simulink library "pathFollowingCtrlAoATurb_cl"  (R2022a)
settings: Solver=VariableStepAuto  StartTime=0.0  StopTime=10.0  RelTol=1e-3
undefined symbols (not defined in the file): env, FLIGHTCONTROLLER, fltCtrl, initializeBussesFromBlock, pthCtrl1, vhcl
libraries: simulink x6, slpidlib x5, velocityAngle_ul x2, stopwatch_ul x1, courseFollowLookAhead_cl x1, ctrlAllocMatrix3Comp_cl x1, eulAng2RotMat_ul x1, angleBtw2Vecs_ul x1, vrlib x1, alphaBeta_ul x1, gnd2TanRotation_ul x1
settings Model: Creator=jldanie5  LastModifiedBy=jacob
settings SolverCC: AlgebraicLoopSolver=TrustRegion
settings DataIOCC: ReturnWorkspaceOutputs=off
settings DebuggingCC: UnconnectedInputMsg=warning  UnconnectedOutputMsg=warning  UnconnectedLineMsg=warning  SFMachineParentedDataDiag=warning  ArithmeticOperatorsInVariantConditions=warning
settings SFSimCC: CustomCodeUndefinedFunction=UseInterfaceOnly

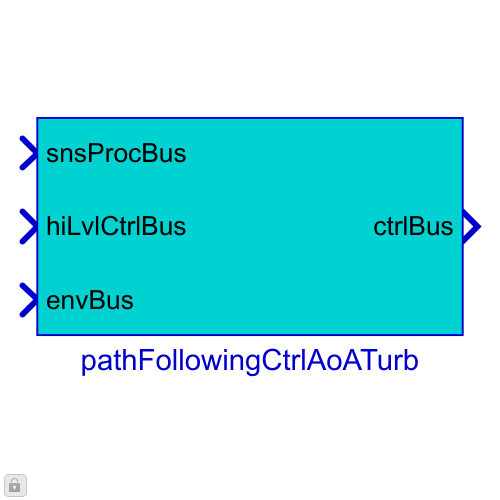
[thumbnail: Simulink's stored preview of the top-level diagram]
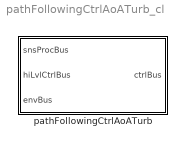
== system pathFollowingCtrlAoATurb_cl ==
  pathFollowingCtrlAoATurb : Subsystem  LoadFcn=initializeBussesFromBlock(gcb)  InitFcn=initializeBussesFromBlock(gcb)  StartFcn=initializeBussesFromBlock(gcb)  VariantControl=strcmpi(FLIGHTCONTROLLER,'pathFollowingControllerManta')  mask{initPosForInitSStar=vhcl.initPosVecGnd.Value, fluidDensity=env.water.density.Value, pathCtrl=pthCtrl1, aeroStruct=vhcl.struct('OCT.aeroSurf')}
      mask prompts: initPosForInitSStar "Initial Position"; fluidDensity "Fluid Density"; pathCtrl "Controller"; aeroStruct "Aerodynamic Structure"
      settings: MinAlgLoopOccurrences=on
      mask DialogControl Container3 Prompt: courseFollow Params
      mask DialogControl Container4 Prompt: setpointToOutput Params

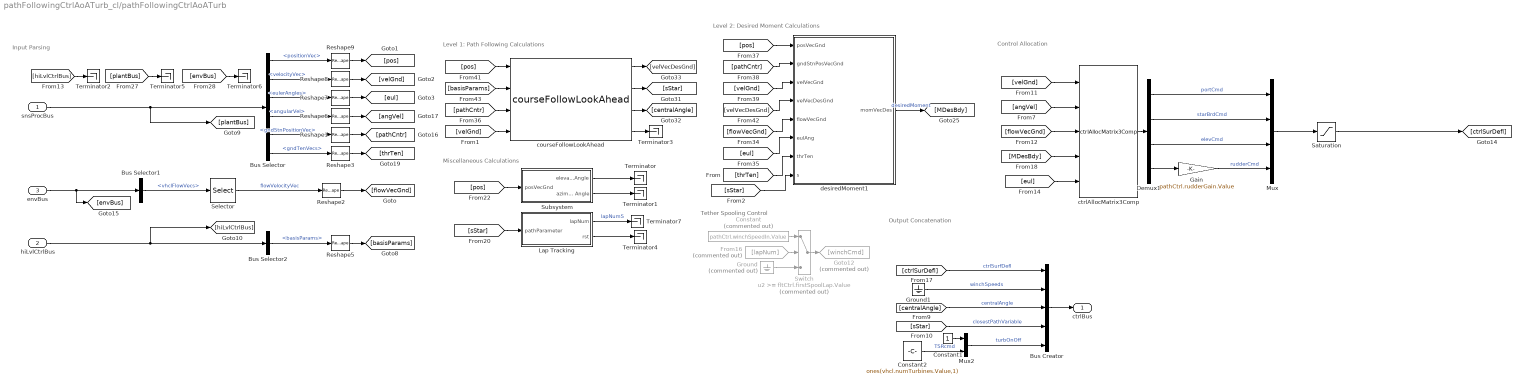
== system pathFollowingCtrlAoATurb_cl/pathFollowingCtrlAoATurb ==
  note: Control Allocation
  note: Miscellaneous Calculations
  note: Output Concatenation
  note: Tether Spooling Control
  note: Input Parsing
  note: Level 1: Path Following Calculations
  note: Level 2: Desired Moment Calculations
  snsProcBus : Inport  OutDataTypeStr=Bus: sensorsProcessingBus
  hiLvlCtrlBus : Inport  Port=2  OutDataTypeStr=Bus: hiLvlCtrlBus
  envBus : Inport  Port=3  OutDataTypeStr=Bus: envBus
  Bus Creator : BusCreator  Inputs=5
  Bus Selector : BusSelector  OutputSignals=positionVec,velocityVec,eulerAngles,angularVel,gndStnPositionVec,gndTenVecs
  Bus Selector1 : BusSelector  OutputSignals=vhclFlowVecs
  Bus Selector2 : BusSelector  OutputSignals=basisParams
  Constant : Constant  Commented=on  Value=pathCtrl.winchSpeedIn.Value
  Constant1 : Constant
  Constant2 : Constant  Value=ones(vhcl.numTurbines.Value,1)
  Demux1 : Demux
  From16 : From  Commented=on  GotoTag=lapNum
  Gain : Gain  Gain=pathCtrl.rudderGain.Value
  Goto12 : Goto  Commented=on  GotoTag=winchCmd
  Ground : Ground  Commented=on
  Ground1 : Ground
  Lap Tracking : Subsystem
  Mux : Mux
  Mux2 : Mux  Inputs=2
  Reshape{1..3,5..9} (8 alike) : Reshape  OutputDimensionality=Column vector (2-D)
  Saturation : Saturate  UpperLimit=30  LowerLimit=-30
  Selector : Selector  NumberOfDimensions=2  InputPortWidth=3  IndexOptions=Select all,Index vector (dialog)  Indices=[1 3],5  OutputSizes=1,1
  Subsystem : Subsystem
  Switch : Switch  Commented=on  Threshold=fltCtrl.firstSpoolLap.Value  SaturateOnIntegerOverflow=off  InputSameDT=off
  Terminator{,1..7} (8 alike) : Terminator
  courseFollowLookAhead : courseFollowLookAhead_cl/courseFollowLookAhead  SystemSampleTime=-1  VariantActivationTime=update diagram  Latency=0  AutoFrameSizeCalculation=off
  ctrlAllocMatrix3Comp : ctrlAllocMatrix3Comp_cl/ctrlAllocMatrix3Comp  aeroStruct=vhcl.struct('OCT.aeroSurf')  fluidDensity=fluidDensity  arms=vhcl.struct('OCT.thrAttch')
  desiredMoment1 : Subsystem
  ctrlBus : Outport  OutDataTypeStr=Bus: fltCtrlBus  VectorParamsAs1DForOutWhenUnconnected=off
  wires:
  Bus Selector/6 -> Reshape3/1  "<gndTenVecs>"
  Reshape3/1 -> [thrTen]
  snsProcBus/1 -> [plantBus], Bus Selector/1
  Bus Selector/2 -> Reshape8/1  "<velocityVec>"
  Bus Selector/1 -> Reshape9/1  "<positionVec>"
  Bus Selector/3 -> Reshape7/1  "<eulerAngles>"
  Bus Creator/1 -> ctrlBus/1
  Ground1/1 -> Bus Creator/2  "winchSpeeds"
  hiLvlCtrlBus/1 -> [hiLvlCtrlBus], Bus Selector2/1
  [centralAngle] -> Bus Creator/3  "centralAngle"
  [sStar] -> Bus Creator/4  "closestPathVariable"
  Bus Selector/4 -> Reshape6/1  "<angularVel>"
  [angVel] -> ctrlAllocMatrix3Comp/2
  [velGnd] -> ctrlAllocMatrix3Comp/1
  [flowVecGnd] -> ctrlAllocMatrix3Comp/3
  Demux1/1 -> Mux/1  "portCmd"
  Demux1/2 -> Mux/2  "starBrdCmd"
  [MDesBdy] -> ctrlAllocMatrix3Comp/4
  [ctrlSurDefl] -> Bus Creator/1  "ctrlSurfDefl"
  Bus Selector2/1 -> Reshape5/1  "<basisParams>"
  Reshape5/1 -> [basisParams]
  Reshape2/1 -> [flowVecGnd]
  Reshape6/1 -> [angVel]
  Reshape7/1 -> [eul]
  Reshape8/1 -> [velGnd]
  Reshape9/1 -> [pos]
  [eul] -> ctrlAllocMatrix3Comp/5
  Selector/1 -> Reshape2/1  "flowVelocityVec"
  envBus/1 -> [envBus], Bus Selector1/1
  Bus Selector1/1 -> Selector/1  "<vhclFlowVecs>"
  Reshape1/1 -> [pathCntr]
  Bus Selector/5 -> Reshape1/1  "<gndStnPositionVec>"
  Demux1/4 -> Gain/1
  [pos] -> Subsystem/1(posVecGnd)
  Subsystem/1(elevationAngle) -> Terminator/1
  Subsystem/2(azimuth Angle) -> Terminator1/1
  [sStar] -> Lap Tracking/1(pathParameter)
  Lap Tracking/2(rst) -> Terminator4/1
  Lap Tracking/1(lapNum) -> Terminator7/1  "lapNumS"
  [plantBus] -> Terminator5/1
  [envBus] -> Terminator6/1
  Switch/1 -> Goto12/1
  From16/1 -> Switch/2
  Constant/1 -> Switch/1
  Ground/1 -> Switch/3
  ctrlAllocMatrix3Comp/1 -> Demux1/1
  Gain/1 -> Mux/4  "rudderCmd"
  [hiLvlCtrlBus] -> Terminator2/1
  Mux2/1 -> Bus Creator/5  "turbOnOff"
  Constant1/1 -> Mux2/1
  Constant2/1 -> Mux2/2  "TSRcmd"
  [velVecDesGnd] -> desiredMoment1/4(velVecDesGnd)
  [velGnd] -> desiredMoment1/3(velVecGnd)
  [eul] -> desiredMoment1/6(eulAng)
  [basisParams] -> courseFollowLookAhead/2
  [pathCntr] -> desiredMoment1/2(gndStnPosVecGnd)
  courseFollowLookAhead/2 -> [sStar]
  [pos] -> desiredMoment1/1(posVecGnd)
  [pathCntr] -> courseFollowLookAhead/3
  desiredMoment1/1(momVecDes) -> [MDesBdy]  "desiredMoment"
  [pos] -> courseFollowLookAhead/1
  courseFollowLookAhead/3 -> [centralAngle]
  courseFollowLookAhead/4 -> Terminator3/1
  courseFollowLookAhead/1 -> [velVecDesGnd]
  [flowVecGnd] -> desiredMoment1/5(flowVecGnd)
  [thrTen] -> desiredMoment1/7(thrTen)
  [velGnd] -> courseFollowLookAhead/4
  Saturation/1 -> [ctrlSurDefl]
  Mux/1 -> Saturation/1
  Demux1/3 -> Mux/3  "elevCmd"
  [sStar] -> desiredMoment1/8(s)

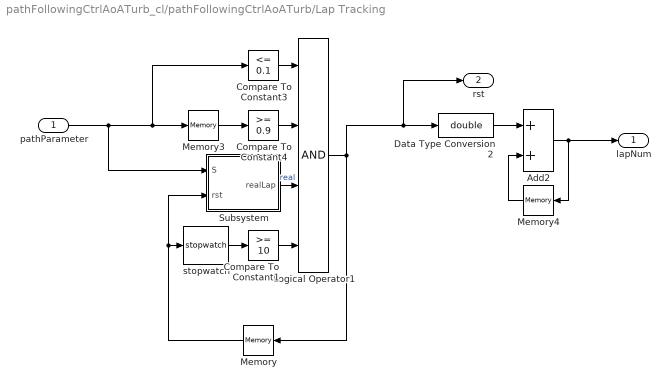
== system pathFollowingCtrlAoATurb_cl/pathFollowingCtrlAoATurb/Lap Tracking ==
  pathParameter : Inport
  Add2 : Sum
  Compare To Constant1 : simulink/Logic and Bit Operations/Compare To Constant  relop=>=  const=10  OutDataTypeStr=boolean
  Compare To Constant3 : simulink/Logic and Bit Operations/Compare To Constant  relop=<=  const=0.1  OutDataTypeStr=boolean
  Compare To Constant4 : simulink/Logic and Bit Operations/Compare To Constant  relop=>=  const=0.9  OutDataTypeStr=boolean
  Data Type Conversion2 : DataTypeConversion  OutDataTypeStr=double  SaturateOnIntegerOverflow=off  RndMeth=Floor
  Logical Operator1 : Logic  Inputs=4  AllPortsSameDT=off  OutDataTypeStr=boolean
  Memory : Memory  InitialCondition=false
  Memory3 : Memory
  Memory4 : Memory
  Subsystem : Subsystem
  stopwatch : stopwatch_ul/stopwatch  SystemSampleTime=-1  VariantActivationTime=update diagram  Latency=0  AutoFrameSizeCalculation=off
  lapNum : Outport  VectorParamsAs1DForOutWhenUnconnected=off
  rst : Outport  Port=2  VectorParamsAs1DForOutWhenUnconnected=off
  wires:
  Compare To Constant3/1 -> Logical Operator1/1
  Memory3/1 -> Compare To Constant4/1
  Data Type Conversion2/1 -> Add2/1
  Logical Operator1/1 -> rst/1, Data Type Conversion2/1, Memory/1
  Memory4/1 -> Add2/2
  Add2/1 -> lapNum/1, Memory4/1
  Compare To Constant4/1 -> Logical Operator1/2
  pathParameter/1 -> Subsystem/1(S), Compare To Constant3/1, Memory3/1
  stopwatch/1 -> Compare To Constant1/1
  Memory/1 -> Subsystem/2(rst), stopwatch/1
  Compare To Constant1/1 -> Logical Operator1/4
  Subsystem/1(realLap) -> Logical Operator1/3  "real"

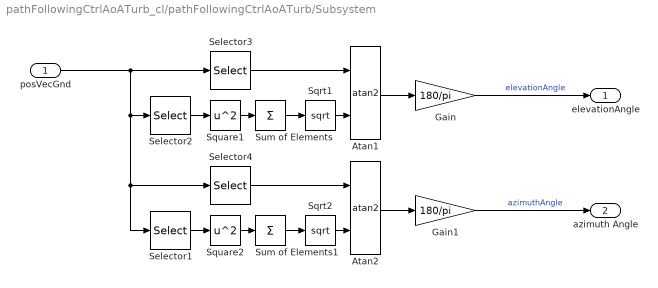
== system pathFollowingCtrlAoATurb_cl/pathFollowingCtrlAoATurb/Subsystem ==
  posVecGnd : Inport
  Atan1 : Trigonometry  Operator=atan2
  Atan2 : Trigonometry  Operator=atan2
  Gain : Gain  Gain=180/pi
  Gain1 : Gain  Gain=180/pi
  Selector1 : Selector  InputPortWidth=3  IndexOptions=Index vector (dialog)  Indices=1  OutputSizes=1
  Selector2 : Selector  InputPortWidth=3  IndexOptions=Index vector (dialog)  Indices=[1 2]  OutputSizes=1
  Selector3 : Selector  InputPortWidth=3  IndexOptions=Index vector (dialog)  Indices=3  OutputSizes=1
  Selector4 : Selector  InputPortWidth=3  IndexOptions=Index vector (dialog)  Indices=2  OutputSizes=1
  Sqrt1 : Sqrt
  Sqrt2 : Sqrt
  Square1 : Math  Operator=square  SignedPower=on
  Square2 : Math  Operator=square  SignedPower=on
  Sum of Elements : Sum  Inputs=+
  Sum of Elements1 : Sum  Inputs=+
  elevationAngle : Outport
  azimuth Angle : Outport  Port=2
  wires:
  Sqrt1/1 -> Atan1/2
  Square1/1 -> Sum of Elements/1
  Selector3/1 -> Atan1/1
  Sum of Elements/1 -> Sqrt1/1
  Atan1/1 -> Gain/1
  Selector2/1 -> Square1/1
  Gain/1 -> elevationAngle/1  "elevationAngle"
  Atan2/1 -> Gain1/1
  Square2/1 -> Sum of Elements1/1
  Sum of Elements1/1 -> Sqrt2/1
  Selector1/1 -> Square2/1
  posVecGnd/1 -> Selector1/1, Selector4/1, Selector2/1, Selector3/1
  Sqrt2/1 -> Atan2/2
  Selector4/1 -> Atan2/1
  Gain1/1 -> azimuth Angle/1  "azimuthAngle"

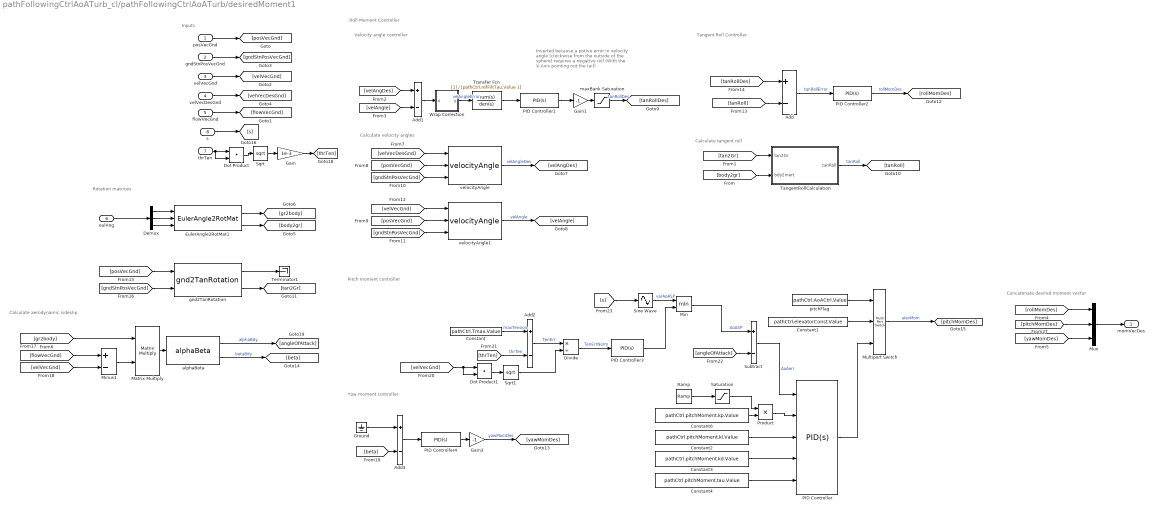
== system pathFollowingCtrlAoATurb_cl/pathFollowingCtrlAoATurb/desiredMoment1 ==
  note: Roll Moment Controller
  note: Calculate aerodynamic sideslip
  note: Concatenate desired moment vector
  note: Tangent Roll Controller
  note: Calculate tangent roll
  note: Calculate velocity angles
  note: Rotation matrices
  note: Inputs
  note: Velocity angle controller
  note: Inverted because a potive error
      | in velocity angle (clockwise from the
      | outside of the sphere) requires a negative
      | roll (With the X-Axis pointing out the tail)
  note: Pitch moment controller
  note: Yaw moment controller
  posVecGnd : Inport
  gndStnPosVecGnd : Inport  Port=2
  velVecGnd : Inport  Port=3
  velVecDesGnd : Inport  Port=4
  flowVecGnd : Inport  Port=5
  eulAng : Inport  Port=6
  thrTen : Inport  Port=7
  s : Inport  Port=8
  Add{,1..3} (4 alike) : Sum  Inputs=+-
  Constant : Constant  Value=pathCtrl.Tmax.Value
  Constant1 : Constant  Value=pathCtrl.elevatorConst.Value
  Constant2 : Constant  Value=pathCtrl.pitchMoment.ki.Value
  Constant3 : Constant  Value=pathCtrl.pitchMoment.kd.Value
  Constant4 : Constant  Value=pathCtrl.pitchMoment.tau.Value
  Constant6 : Constant  Value=pathCtrl.pitchMoment.kp.Value
  Demux : Demux  Outputs=3
  Divide : Product  Inputs=*/
  Dot Product : DotProduct  OutDataTypeStr=Inherit: Inherit via internal rule
  Dot Product1 : DotProduct  OutDataTypeStr=Inherit: Inherit via internal rule
  EulerAngle2RotMat1 : eulAng2RotMat_ul/EulerAngle2RotMat  SystemSampleTime=-1  VariantActivationTime=update diagram  Latency=0  AutoFrameSizeCalculation=off
  Gain : Gain  Gain=1e-3
  Gain1 : Gain  Gain=-1
  Gain3 : Gain  Gain=-1
  Ground : Ground
  Matrix Multiply : Product  Multiplication=Matrix(*)
  Min : MinMax  Inputs=2
  Minus1 : Sum  Inputs=+-
  Multiport Switch : MultiPortSwitch  DataPortOrder=Specify indices  Inputs=2  DataPortIndices={0,1}  SaturateOnIntegerOverflow=off  InputSameDT=off
  Mux : Mux  Inputs=3
  PID Controller : slpidlib/PID Controller  Controller=PID  Form=Parallel  TimeDomain=Continuous-time  UseExternalTs=off  SampleTime=-1  IntegratorMethod=Forward Euler  FilterMethod=Forward Euler  ControllerParametersSource=external  P=pathCtrl.pitchMoment.kp.Value  I=pathCtrl.pitchMoment.ki.Value  UseKiTs=off  D=pathCtrl.pitchMoment.kd.Value  N=1/pathCtrl.pitchMoment.tau.Value  UseFilter=on  TunerSelectOption=Transfer Function Based (PID Tuner App)  InitialConditionSource=internal  InitialConditionForIntegrator=0  InitialConditionForFilter=0  DifferentiatorICPrevScaledInput=0  ExternalReset=none  TrackingMode=off  Kt=1  LimitOutput=off  SatLimitsSource=internal  UpperSaturationLimit=inf  LowerSaturationLimit=-100  LinearizeAsGain=on  AntiWindupMode=clamping  Kb=1  POutMin=[]  POutMax=[]  IOutMin=[]  IOutMax=[]  DOutMin=[]  DOutMax=[]  NOutMin=[]  NOutMax=[]  SumOutMin=[]  SumOutMax=[]  SaturationOutMin=[]  SaturationOutMax=[]  PParamMin=[]  PParamMax=[]  IParamMin=[]  IParamMax=[]  DParamMin=[]  DParamMax=[]  NParamMin=[]  NParamMax=[]  KbParamMin=[]  KbParamMax=[]  KtParamMin=[]  KtParamMax=[]  KbOutMin=[]  KbOutMax=[]  KtOutMin=[]  KtOutMax=[]  IntegratorOutMin=[]  IntegratorOutMax=[]  FilterOutMin=[]  FilterOutMax=[]  SumI1OutMin=[]  SumI1OutMax=[]  SumI2OutMin=[]  SumI2OutMax=[]  SumI3OutMin=[]  SumI3OutMax=[]  SumI4OutMin=[]  SumI4OutMax=[]  SumDOutMin=[]  SumDOutMax=[]  DifferentiatorOutMin=[]  DifferentiatorOutMax=[]  FilterDiffOutCoefMin=[]  FilterDiffOutCoefMax=[]  ReciprocalOutMin=[]  ReciprocalOutMax=[]  SumDenOutMin=[]  SumDenOutMax=[]  SumNumOutMin=[]  SumNumOutMax=[]  DivideOutMin=[]  DivideOutMax=[]  UdiffTsProdOutMin=[]  UdiffTsProdOutMax=[]  NTsProdOutMin=[]  NTsProdOutMax=[]  UintegralTsProdOutMin=[]  UintegralTsProdOutMax=[]  UngainTsProdOutMin=[]  UngainTsProdOutMax=[]  ClampingZeroOutDataTypeStr=Inherit: Inherit via back propagation  ClampingZeroOutMin=[]  ClampingZeroOutMax=[]  FilterDenConstantOutDataTypeStr=Inherit: Inherit via back propagation  FilterDenConstantOutMin=[]  FilterDenConstantOutMax=[]  PCopyOutDataTypeStr=Inherit: Inherit via back propagation  PCopyOutMin=[]  PCopyOutMax=[]  NCopyOutDataTypeStr=Inherit: Inherit via back propagation  NCopyOutMin=[]  NCopyOutMax=[]  IntegratorContinuousStateAttributes=''  IntegratorStateMustResolveToSignalObject=off  IntegratorRTWStateStorageClass=Auto  FilterContinuousStateAttributes=''  FilterStateMustResolveToSignalObject=off  FilterRTWStateStorageClass=Auto  ParallelPVariant=ExternalParameters  IdealPVariant=Disabled  IVariant=ExternalParameters  DVariant=ExternalParameters  IntegratorVariant=Continuous  SatVariant=Disabled  AWVariant=Passthrough  PCopyVariant=Disabled  TRVariant=Disabled  FdbkBlocksVariant=Forward  IdealPFdbkVariant=Disabled  SatFdbkVariant=Disabled  DerivativeFilterVariant=ContFilter  NVariant=ExternalParameters  NCopyVariant=Disabled  FilterICVariant=InternalICsFilter  IntegratorICVariant=InternalICs  ExternalResetVariant=Disabled  TRSumVariant=Passthrough  SumFdbkVariant=Disabled  SumVariant=Sum_PID  TsampFilterVariant=InternalTs  TsampNgainVariant=Passthrough  TsampIntegralVariant=Passthrough  ExternalSaturationOutDataTypeStr=Inherit: Same as second input  aMode=0
  PID Controller1 : slpidlib/PID Controller  Controller=PID  Form=Parallel  TimeDomain=Continuous-time  UseExternalTs=off  SampleTime=-1  IntegratorMethod=Forward Euler  FilterMethod=Forward Euler  ControllerParametersSource=internal  P=pathCtrl.tanRoll.kp.Value  I=pathCtrl.tanRoll.ki.Value  UseKiTs=off  D=pathCtrl.tanRoll.kd.Value  N=1/pathCtrl.tanRoll.tau.Value  UseFilter=on  TunerSelectOption=Transfer Function Based (PID Tuner App)  InitialConditionSource=internal  InitialConditionForIntegrator=0  InitialConditionForFilter=0  DifferentiatorICPrevScaledInput=0  ExternalReset=none  TrackingMode=off  Kt=1  LimitOutput=off  SatLimitsSource=internal  UpperSaturationLimit=inf  LowerSaturationLimit=-100  LinearizeAsGain=on  AntiWindupMode=clamping  Kb=1  POutMin=[]  POutMax=[]  IOutMin=[]  IOutMax=[]  DOutMin=[]  DOutMax=[]  NOutMin=[]  NOutMax=[]  SumOutMin=[]  SumOutMax=[]  SaturationOutMin=[]  SaturationOutMax=[]  PParamMin=[]  PParamMax=[]  IParamMin=[]  IParamMax=[]  DParamMin=[]  DParamMax=[]  NParamMin=[]  NParamMax=[]  KbParamMin=[]  KbParamMax=[]  KtParamMin=[]  KtParamMax=[]  KbOutMin=[]  KbOutMax=[]  KtOutMin=[]  KtOutMax=[]  IntegratorOutMin=[]  IntegratorOutMax=[]  FilterOutMin=[]  FilterOutMax=[]  SumI1OutMin=[]  SumI1OutMax=[]  SumI2OutMin=[]  SumI2OutMax=[]  SumI3OutMin=[]  SumI3OutMax=[]  SumI4OutMin=[]  SumI4OutMax=[]  SumDOutMin=[]  SumDOutMax=[]  DifferentiatorOutMin=[]  DifferentiatorOutMax=[]  FilterDiffOutCoefMin=[]  FilterDiffOutCoefMax=[]  ReciprocalOutMin=[]  ReciprocalOutMax=[]  SumDenOutMin=[]  SumDenOutMax=[]  SumNumOutMin=[]  SumNumOutMax=[]  DivideOutMin=[]  DivideOutMax=[]  UdiffTsProdOutMin=[]  UdiffTsProdOutMax=[]  NTsProdOutMin=[]  NTsProdOutMax=[]  UintegralTsProdOutMin=[]  UintegralTsProdOutMax=[]  UngainTsProdOutMin=[]  UngainTsProdOutMax=[]  ClampingZeroOutDataTypeStr=Inherit: Inherit via back propagation  ClampingZeroOutMin=[]  ClampingZeroOutMax=[]  FilterDenConstantOutDataTypeStr=Inherit: Inherit via back propagation  FilterDenConstantOutMin=[]  FilterDenConstantOutMax=[]  PCopyOutDataTypeStr=Inherit: Inherit via back propagation  PCopyOutMin=[]  PCopyOutMax=[]  NCopyOutDataTypeStr=Inherit: Inherit via back propagation  NCopyOutMin=[]  NCopyOutMax=[]  IntegratorContinuousStateAttributes=''  IntegratorStateMustResolveToSignalObject=off  IntegratorRTWStateStorageClass=Auto  FilterContinuousStateAttributes=''  FilterStateMustResolveToSignalObject=off  FilterRTWStateStorageClass=Auto  ParallelPVariant=InternalParameters  IdealPVariant=Disabled  IVariant=InternalParameters  DVariant=InternalParameters  IntegratorVariant=Continuous  SatVariant=Disabled  AWVariant=Passthrough  PCopyVariant=Disabled  TRVariant=Disabled  FdbkBlocksVariant=Forward  IdealPFdbkVariant=Disabled  SatFdbkVariant=Disabled  DerivativeFilterVariant=ContFilter  NVariant=InternalParameters  NCopyVariant=Disabled  FilterICVariant=InternalICsFilter  IntegratorICVariant=InternalICs  ExternalResetVariant=Disabled  TRSumVariant=Passthrough  SumFdbkVariant=Disabled  SumVariant=Sum_PID  TsampFilterVariant=InternalTs  TsampNgainVariant=Passthrough  TsampIntegralVariant=Passthrough  ExternalSaturationOutDataTypeStr=Inherit: Same as second input  aMode=0
  PID Controller2 : slpidlib/PID Controller  Controller=PID  Form=Parallel  TimeDomain=Continuous-time  UseExternalTs=off  SampleTime=-1  IntegratorMethod=Forward Euler  FilterMethod=Forward Euler  ControllerParametersSource=internal  P=pathCtrl.rollMoment.kp.Value  I=pathCtrl.rollMoment.ki.Value  UseKiTs=off  D=pathCtrl.rollMoment.kd.Value  N=1/pathCtrl.rollMoment.tau.Value  UseFilter=on  TunerSelectOption=Transfer Function Based (PID Tuner App)  InitialConditionSource=internal  InitialConditionForIntegrator=0  InitialConditionForFilter=0  DifferentiatorICPrevScaledInput=0  ExternalReset=none  TrackingMode=off  Kt=1  LimitOutput=off  SatLimitsSource=internal  UpperSaturationLimit=inf  LowerSaturationLimit=-100  LinearizeAsGain=on  AntiWindupMode=clamping  Kb=1  POutMin=[]  POutMax=[]  IOutMin=[]  IOutMax=[]  DOutMin=[]  DOutMax=[]  NOutMin=[]  NOutMax=[]  SumOutMin=[]  SumOutMax=[]  SaturationOutMin=[]  SaturationOutMax=[]  PParamMin=[]  PParamMax=[]  IParamMin=[]  IParamMax=[]  DParamMin=[]  DParamMax=[]  NParamMin=[]  NParamMax=[]  KbParamMin=[]  KbParamMax=[]  KtParamMin=[]  KtParamMax=[]  KbOutMin=[]  KbOutMax=[]  KtOutMin=[]  KtOutMax=[]  IntegratorOutMin=[]  IntegratorOutMax=[]  FilterOutMin=[]  FilterOutMax=[]  SumI1OutMin=[]  SumI1OutMax=[]  SumI2OutMin=[]  SumI2OutMax=[]  SumI3OutMin=[]  SumI3OutMax=[]  SumI4OutMin=[]  SumI4OutMax=[]  SumDOutMin=[]  SumDOutMax=[]  DifferentiatorOutMin=[]  DifferentiatorOutMax=[]  FilterDiffOutCoefMin=[]  FilterDiffOutCoefMax=[]  ReciprocalOutMin=[]  ReciprocalOutMax=[]  SumDenOutMin=[]  SumDenOutMax=[]  SumNumOutMin=[]  SumNumOutMax=[]  DivideOutMin=[]  DivideOutMax=[]  UdiffTsProdOutMin=[]  UdiffTsProdOutMax=[]  NTsProdOutMin=[]  NTsProdOutMax=[]  UintegralTsProdOutMin=[]  UintegralTsProdOutMax=[]  UngainTsProdOutMin=[]  UngainTsProdOutMax=[]  ClampingZeroOutDataTypeStr=Inherit: Inherit via back propagation  ClampingZeroOutMin=[]  ClampingZeroOutMax=[]  FilterDenConstantOutDataTypeStr=Inherit: Inherit via back propagation  FilterDenConstantOutMin=[]  FilterDenConstantOutMax=[]  PCopyOutDataTypeStr=Inherit: Inherit via back propagation  PCopyOutMin=[]  PCopyOutMax=[]  NCopyOutDataTypeStr=Inherit: Inherit via back propagation  NCopyOutMin=[]  NCopyOutMax=[]  IntegratorContinuousStateAttributes=''  IntegratorStateMustResolveToSignalObject=off  IntegratorRTWStateStorageClass=Auto  FilterContinuousStateAttributes=''  FilterStateMustResolveToSignalObject=off  FilterRTWStateStorageClass=Auto  ParallelPVariant=InternalParameters  IdealPVariant=Disabled  IVariant=InternalParameters  DVariant=InternalParameters  IntegratorVariant=Continuous  SatVariant=Disabled  AWVariant=Passthrough  PCopyVariant=Disabled  TRVariant=Disabled  FdbkBlocksVariant=Forward  IdealPFdbkVariant=Disabled  SatFdbkVariant=Disabled  DerivativeFilterVariant=ContFilter  NVariant=InternalParameters  NCopyVariant=Disabled  FilterICVariant=InternalICsFilter  IntegratorICVariant=InternalICs  ExternalResetVariant=Disabled  TRSumVariant=Passthrough  SumFdbkVariant=Disabled  SumVariant=Sum_PID  TsampFilterVariant=InternalTs  TsampNgainVariant=Passthrough  TsampIntegralVariant=Passthrough  ExternalSaturationOutDataTypeStr=Inherit: Same as second input  aMode=0
  PID Controller3 : slpidlib/PID Controller  Controller=PID  Form=Parallel  TimeDomain=Continuous-time  UseExternalTs=off  SampleTime=-1  IntegratorMethod=Forward Euler  FilterMethod=Forward Euler  ControllerParametersSource=internal  P=pathCtrl.alphaCtrl.kp.Value  I=pathCtrl.alphaCtrl.ki.Value  UseKiTs=off  D=pathCtrl.alphaCtrl.kd.Value  N=1/pathCtrl.alphaCtrl.tau.Value  UseFilter=on  TunerSelectOption=Transfer Function Based (PID Tuner App)  InitialConditionSource=internal  InitialConditionForIntegrator=0  InitialConditionForFilter=0  DifferentiatorICPrevScaledInput=0  ExternalReset=none  TrackingMode=off  Kt=1  LimitOutput=on  SatLimitsSource=internal  UpperSaturationLimit=pathCtrl.AoAConst.Value  LowerSaturationLimit=pathCtrl.AoAmin.Value  LinearizeAsGain=on  AntiWindupMode=clamping  Kb=1  POutMin=[]  POutMax=[]  IOutMin=[]  IOutMax=[]  DOutMin=[]  DOutMax=[]  NOutMin=[]  NOutMax=[]  SumOutMin=[]  SumOutMax=[]  SaturationOutMin=[]  SaturationOutMax=[]  PParamMin=[]  PParamMax=[]  IParamMin=[]  IParamMax=[]  DParamMin=[]  DParamMax=[]  NParamMin=[]  NParamMax=[]  KbParamMin=[]  KbParamMax=[]  KtParamMin=[]  KtParamMax=[]  KbOutMin=[]  KbOutMax=[]  KtOutMin=[]  KtOutMax=[]  IntegratorOutMin=[]  IntegratorOutMax=[]  FilterOutMin=[]  FilterOutMax=[]  SumI1OutMin=[]  SumI1OutMax=[]  SumI2OutMin=[]  SumI2OutMax=[]  SumI3OutMin=[]  SumI3OutMax=[]  SumI4OutMin=[]  SumI4OutMax=[]  SumDOutMin=[]  SumDOutMax=[]  DifferentiatorOutMin=[]  DifferentiatorOutMax=[]  FilterDiffOutCoefMin=[]  FilterDiffOutCoefMax=[]  ReciprocalOutMin=[]  ReciprocalOutMax=[]  SumDenOutMin=[]  SumDenOutMax=[]  SumNumOutMin=[]  SumNumOutMax=[]  DivideOutMin=[]  DivideOutMax=[]  UdiffTsProdOutMin=[]  UdiffTsProdOutMax=[]  NTsProdOutMin=[]  NTsProdOutMax=[]  UintegralTsProdOutMin=[]  UintegralTsProdOutMax=[]  UngainTsProdOutMin=[]  UngainTsProdOutMax=[]  ClampingZeroOutDataTypeStr=Inherit: Inherit via back propagation  ClampingZeroOutMin=[]  ClampingZeroOutMax=[]  FilterDenConstantOutDataTypeStr=Inherit: Inherit via back propagation  FilterDenConstantOutMin=[]  FilterDenConstantOutMax=[]  PCopyOutDataTypeStr=Inherit: Inherit via back propagation  PCopyOutMin=[]  PCopyOutMax=[]  NCopyOutDataTypeStr=Inherit: Inherit via back propagation  NCopyOutMin=[]  NCopyOutMax=[]  IntegratorContinuousStateAttributes=''  IntegratorStateMustResolveToSignalObject=off  IntegratorRTWStateStorageClass=Auto  FilterContinuousStateAttributes=''  FilterStateMustResolveToSignalObject=off  FilterRTWStateStorageClass=Auto  ParallelPVariant=InternalParameters  IdealPVariant=Disabled  IVariant=InternalParameters  DVariant=InternalParameters  IntegratorVariant=Continuous  SatVariant=Enabled  AWVariant=ContClampingParallel  PCopyVariant=Disabled  TRVariant=Disabled  FdbkBlocksVariant=Forward  IdealPFdbkVariant=Disabled  SatFdbkVariant=Disabled  DerivativeFilterVariant=ContFilter  NVariant=InternalParameters  NCopyVariant=Disabled  FilterICVariant=InternalICsFilter  IntegratorICVariant=InternalICs  ExternalResetVariant=Disabled  TRSumVariant=Passthrough  SumFdbkVariant=Disabled  SumVariant=Sum_PID  TsampFilterVariant=InternalTs  TsampNgainVariant=Passthrough  TsampIntegralVariant=Passthrough  ExternalSaturationOutDataTypeStr=Inherit: Same as second input  aMode=0
  PID Controller4 : slpidlib/PID Controller  Controller=PID  Form=Parallel  TimeDomain=Continuous-time  UseExternalTs=off  SampleTime=-1  IntegratorMethod=Forward Euler  FilterMethod=Forward Euler  ControllerParametersSource=internal  P=pathCtrl.yawMoment.kp.Value  I=pathCtrl.yawMoment.ki.Value  UseKiTs=off  D=pathCtrl.yawMoment.kd.Value  N=1/pathCtrl.yawMoment.tau.Value  UseFilter=on  TunerSelectOption=Transfer Function Based (PID Tuner App)  InitialConditionSource=internal  InitialConditionForIntegrator=0  InitialConditionForFilter=0  DifferentiatorICPrevScaledInput=0  ExternalReset=none  TrackingMode=off  Kt=1  LimitOutput=off  SatLimitsSource=internal  UpperSaturationLimit=inf  LowerSaturationLimit=-100  LinearizeAsGain=on  AntiWindupMode=clamping  Kb=1  POutMin=[]  POutMax=[]  IOutMin=[]  IOutMax=[]  DOutMin=[]  DOutMax=[]  NOutMin=[]  NOutMax=[]  SumOutMin=[]  SumOutMax=[]  SaturationOutMin=[]  SaturationOutMax=[]  PParamMin=[]  PParamMax=[]  IParamMin=[]  IParamMax=[]  DParamMin=[]  DParamMax=[]  NParamMin=[]  NParamMax=[]  KbParamMin=[]  KbParamMax=[]  KtParamMin=[]  KtParamMax=[]  KbOutMin=[]  KbOutMax=[]  KtOutMin=[]  KtOutMax=[]  IntegratorOutMin=[]  IntegratorOutMax=[]  FilterOutMin=[]  FilterOutMax=[]  SumI1OutMin=[]  SumI1OutMax=[]  SumI2OutMin=[]  SumI2OutMax=[]  SumI3OutMin=[]  SumI3OutMax=[]  SumI4OutMin=[]  SumI4OutMax=[]  SumDOutMin=[]  SumDOutMax=[]  DifferentiatorOutMin=[]  DifferentiatorOutMax=[]  FilterDiffOutCoefMin=[]  FilterDiffOutCoefMax=[]  ReciprocalOutMin=[]  ReciprocalOutMax=[]  SumDenOutMin=[]  SumDenOutMax=[]  SumNumOutMin=[]  SumNumOutMax=[]  DivideOutMin=[]  DivideOutMax=[]  UdiffTsProdOutMin=[]  UdiffTsProdOutMax=[]  NTsProdOutMin=[]  NTsProdOutMax=[]  UintegralTsProdOutMin=[]  UintegralTsProdOutMax=[]  UngainTsProdOutMin=[]  UngainTsProdOutMax=[]  ClampingZeroOutDataTypeStr=Inherit: Inherit via back propagation  ClampingZeroOutMin=[]  ClampingZeroOutMax=[]  FilterDenConstantOutDataTypeStr=Inherit: Inherit via back propagation  FilterDenConstantOutMin=[]  FilterDenConstantOutMax=[]  PCopyOutDataTypeStr=Inherit: Inherit via back propagation  PCopyOutMin=[]  PCopyOutMax=[]  NCopyOutDataTypeStr=Inherit: Inherit via back propagation  NCopyOutMin=[]  NCopyOutMax=[]  IntegratorContinuousStateAttributes=''  IntegratorStateMustResolveToSignalObject=off  IntegratorRTWStateStorageClass=Auto  FilterContinuousStateAttributes=''  FilterStateMustResolveToSignalObject=off  FilterRTWStateStorageClass=Auto  ParallelPVariant=InternalParameters  IdealPVariant=Disabled  IVariant=InternalParameters  DVariant=InternalParameters  IntegratorVariant=Continuous  SatVariant=Disabled  AWVariant=Passthrough  PCopyVariant=Disabled  TRVariant=Disabled  FdbkBlocksVariant=Forward  IdealPFdbkVariant=Disabled  SatFdbkVariant=Disabled  DerivativeFilterVariant=ContFilter  NVariant=InternalParameters  NCopyVariant=Disabled  FilterICVariant=InternalICsFilter  IntegratorICVariant=InternalICs  ExternalResetVariant=Disabled  TRSumVariant=Passthrough  SumFdbkVariant=Disabled  SumVariant=Sum_PID  TsampFilterVariant=InternalTs  TsampNgainVariant=Passthrough  TsampIntegralVariant=Passthrough  ExternalSaturationOutDataTypeStr=Inherit: Same as second input  aMode=0
  Product : Product
  Ramp : simulink/Sources/Ramp  slope=0.05  start=100  InitialOutput=0.2
  Saturation : Saturate  UpperLimit=1  LowerLimit=0.2
  Sine Wave : Sin  TimeSource=Use external signal  Amplitude=1*pi/180  Bias=15*pi/180  Frequency=4*pi  Phase=pi/2  SampleTime=0
  Sqrt : Sqrt
  Sqrt1 : Sqrt
  Subtract : Sum  Inputs=+-
  TangentRollCalculation : Subsystem
  Terminator1 : Terminator
  Transfer Fcn : TransferFcn  Denominator=[pathCtrl.refFiltTau.Value 1]
  Wrap Correction : Subsystem
  alphaBeta : alphaBeta_ul/alphaBeta  SystemSampleTime=-1  VariantActivationTime=update diagram  Latency=0  AutoFrameSizeCalculation=off
  gnd2TanRotation : gnd2TanRotation_ul/gnd2TanRotation  SystemSampleTime=-1  VariantActivationTime=update diagram  Latency=0  AutoFrameSizeCalculation=off
  maxBank Saturation : Saturate  UpperLimit=pathCtrl.maxBank.upperLimit.Value  LowerLimit=pathCtrl.maxBank.lowerLimit.Value
  pitchFlag : Constant  Value=pathCtrl.AoACtrl.Value
  velocityAngle : velocityAngle_ul/velocityAngle  SystemSampleTime=-1  VariantActivationTime=update diagram  Latency=0  AutoFrameSizeCalculation=off
  velocityAngle1 : velocityAngle_ul/velocityAngle  SystemSampleTime=-1  VariantActivationTime=update diagram  Latency=0  AutoFrameSizeCalculation=off
  momVecDes : Outport  VectorParamsAs1DForOutWhenUnconnected=off
  wires:
  PID Controller2/1 -> [rollMomDes]  "rollMomDes"
  [rollMomDes] -> Mux/1
  Wrap Correction/1(y) -> Transfer Fcn/1  "velAngleError"
  posVecGnd/1 -> [posVecGnd]
  velVecGnd/1 -> [velVecGnd]
  Add/1 -> PID Controller2/1  "tanRollError"
  Gain1/1 -> maxBank Saturation/1
  maxBank Saturation/1 -> [tanRollDes]  "tanRollDes"
  Add1/1 -> Wrap Correction/1(u)
  flowVecGnd/1 -> [flowVecGnd]
  [tan2Gr] -> TangentRollCalculation/1(tan2Gr)
  TangentRollCalculation/1(tanRoll) -> [tanRoll]  "tanRoll"
  Minus1/1 -> Matrix Multiply/2
  [velVecGnd] -> Minus1/2
  [flowVecGnd] -> Minus1/1
  eulAng/1 -> Demux/1
  Demux/2 -> EulerAngle2RotMat1/2
  EulerAngle2RotMat1/2 -> [body2gr]
  EulerAngle2RotMat1/1 -> [gr2body]
  [body2gr] -> TangentRollCalculation/2(bdy2Inert)
  [gr2body] -> Matrix Multiply/1
  Matrix Multiply/1 -> alphaBeta/1
  alphaBeta/2 -> [beta]  "betaBdy"
  alphaBeta/1 -> [angleOfAttack]  "alphaBdy"
  gndStnPosVecGnd/1 -> [gndStnPosVecGnd]
  velVecDesGnd/1 -> [velVecDesGnd]
  velocityAngle/1 -> [velAngDes]  "velAngleDes"
  velocityAngle1/1 -> [velAngle]  "velAngle"
  [velAngDes] -> Add1/1
  [velAngle] -> Add1/2
  [velVecDesGnd] -> velocityAngle/1
  [posVecGnd] -> velocityAngle/2
  [posVecGnd] -> velocityAngle1/2
  [gndStnPosVecGnd] -> velocityAngle/3
  [gndStnPosVecGnd] -> velocityAngle1/3
  [velVecGnd] -> velocityAngle1/1
  [tanRoll] -> Add/2
  [tanRollDes] -> Add/1
  [posVecGnd] -> gnd2TanRotation/1
  [gndStnPosVecGnd] -> gnd2TanRotation/2
  gnd2TanRotation/2 -> [tan2Gr]
  gnd2TanRotation/1 -> Terminator1/1
  [yawMomDes] -> Mux/3
  PID Controller1/1 -> Gain1/1
  [beta] -> Add3/2
  Ground/1 -> Add3/1
  Add3/1 -> PID Controller4/1
  PID Controller4/1 -> Gain3/1
  [pitchMomDes] -> Mux/2
  Multiport Switch/1 -> [pitchMomDes]  "elevMom"
  pitchFlag/1 -> Multiport Switch/1
  [angleOfAttack] -> Subtract/2
  Constant1/1 -> Multiport Switch/2
  PID Controller/1 -> Multiport Switch/3
  Subtract/1 -> PID Controller/1  "AoAerr"
  thrTen/1 -> Dot Product/2, Dot Product/1
  Sqrt/1 -> Gain/1
  Dot Product/1 -> Sqrt/1
  Gain/1 -> [thrTen]
  [velVecGnd] -> Dot Product1/2, Dot Product1/1
  Dot Product1/1 -> Sqrt1/1
  Demux/1 -> EulerAngle2RotMat1/1
  Demux/3 -> EulerAngle2RotMat1/3
  Mux/1 -> momVecDes/1
  Transfer Fcn/1 -> PID Controller1/1
  [thrTen] -> Add2/2  "thrTen"
  Add2/1 -> Divide/1  "TenErr"
  Sqrt1/1 -> Divide/2
  Constant/1 -> Add2/1  "maxTension"
  Divide/1 -> PID Controller3/1  "TenErrNorm"
  Constant2/1 -> PID Controller/3
  Constant3/1 -> PID Controller/4
  Constant4/1 -> PID Controller/5
  Ramp/1 -> Saturation/1
  Constant6/1 -> Product/2
  Product/1 -> PID Controller/2
  Saturation/1 -> Product/1
  s/1 -> [s]
  [s] -> Sine Wave/1
  Sine Wave/1 -> Min/1  "varAoASP"
  PID Controller3/1 -> Min/2
  Min/1 -> Subtract/1  "AoASP"
  Gain3/1 -> [yawMomDes]  "yawMomDes"

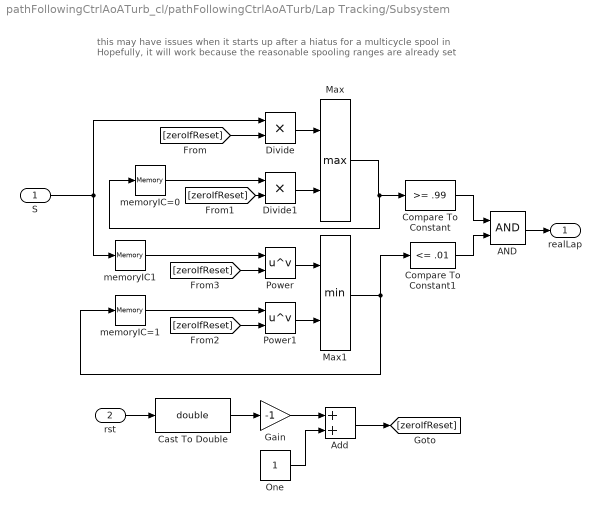
== system pathFollowingCtrlAoATurb_cl/pathFollowingCtrlAoATurb/Lap Tracking/Subsystem ==
  note: this may have issues when it starts up after a hiatus for a multicycle spool in
      | Hopefully, it will work because the reasonable spooling ranges are already set
  S : Inport
  rst : Inport  Port=2
  AND : Logic  AllPortsSameDT=off  OutDataTypeStr=boolean
  Add : Sum
  Cast To Double : DataTypeConversion  OutDataTypeStr=double  SaturateOnIntegerOverflow=off  RndMeth=Floor
  Compare To Constant : simulink/Logic and Bit Operations/Compare To Constant  relop=>=  const=.99  OutDataTypeStr=boolean
  Compare To Constant1 : simulink/Logic and Bit Operations/Compare To Constant  relop=<=  const=.01  OutDataTypeStr=boolean
  Divide : Product  Inputs=**
  Divide1 : Product  Inputs=**
  Gain : Gain  Gain=-1
  Max : MinMax  Function=max  Inputs=2
  Max1 : MinMax  Inputs=2
  One : Constant  OutDataTypeStr=Inherit: Inherit via back propagation
  Power : Math  Operator=pow
  Power1 : Math  Operator=pow
  memoryIC1 : Memory  InitialCondition=1
  memoryIC=0 : Memory
  memoryIC=1 : Memory  InitialCondition=1
  realLap : Outport
  wires:
  Max1/1 -> Compare To Constant1/1, memoryIC=1/1
  rst/1 -> Cast To Double/1
  S/1 -> Divide/1, memoryIC1/1
  Gain/1 -> Add/1
  Add/1 -> [zeroIfReset]
  One/1 -> Add/2
  Divide/1 -> Max/1
  Max/1 -> memoryIC=0/1, Compare To Constant/1
  Power/1 -> Max1/1
  Power1/1 -> Max1/2
  Cast To Double/1 -> Gain/1
  Compare To Constant/1 -> AND/1
  Compare To Constant1/1 -> AND/2
  AND/1 -> realLap/1
  [zeroIfReset] -> Divide/2
  [zeroIfReset] -> Power/2
  [zeroIfReset] -> Divide1/2
  Divide1/1 -> Max/2
  memoryIC=0/1 -> Divide1/1
  [zeroIfReset] -> Power1/2
  memoryIC=1/1 -> Power1/1
  memoryIC1/1 -> Power/1

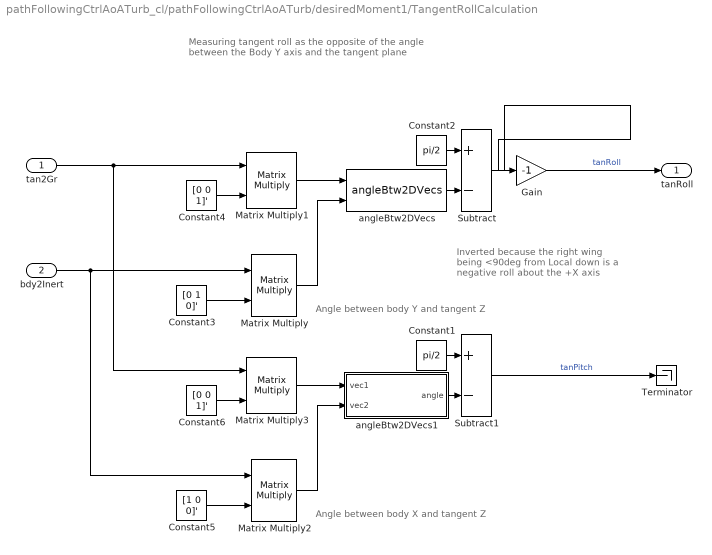
== system pathFollowingCtrlAoATurb_cl/pathFollowingCtrlAoATurb/desiredMoment1/TangentRollCalculation ==
  note: Measuring tangent roll as the opposite
      | of the angle between the Body Y axis
      | and the tangent plane
  note: Angle between body Y and tangent Z
  note: Inverted because the right wing
      | being <90deg from Local down
      | is a negative roll about the +X axis
  note: Angle between body X and tangent Z
  tan2Gr : Inport
  bdy2Inert : Inport  Port=2
  Constant1 : Constant  Value=pi/2
  Constant2 : Constant  Value=pi/2
  Constant3 : Constant  Value=[0 1 0]'
  Constant4 : Constant  Value=[0 0 1]'
  Constant5 : Constant  Value=[1 0 0]'
  Constant6 : Constant  Value=[0 0 1]'
  Gain : Gain  Gain=-1
  Matrix Multiply{,1..3} (4 alike) : Product  Multiplication=Matrix(*)
  Subtract : Sum  Inputs=+-
  Subtract1 : Sum  Inputs=+-
  Terminator : Terminator
  angleBtw2DVecs : angleBtw2Vecs_ul/angleBtw2DVecs  SystemSampleTime=-1  VariantActivationTime=update diagram  Latency=0  AutoFrameSizeCalculation=off
  angleBtw2DVecs1 : Subsystem
  tanRoll : Outport  VectorParamsAs1DForOutWhenUnconnected=off
  wires:
  Subtract/1 -> Gain/1
  Constant3/1 -> Matrix Multiply/2
  angleBtw2DVecs/1 -> Subtract/2
  Constant2/1 -> Subtract/1
  Matrix Multiply1/1 -> angleBtw2DVecs/1
  Constant4/1 -> Matrix Multiply1/2
  Matrix Multiply/1 -> angleBtw2DVecs/2
  Gain/1 -> tanRoll/1  "tanRoll"
  bdy2Inert/1 -> Matrix Multiply2/1, Matrix Multiply/1
  Subtract1/1 -> Terminator/1  "tanPitch"
  tan2Gr/1 -> Matrix Multiply3/1, Matrix Multiply1/1
  Matrix Multiply2/1 -> angleBtw2DVecs1/2(vec2)
  Constant6/1 -> Matrix Multiply3/2
  Matrix Multiply3/1 -> angleBtw2DVecs1/1(vec1)
  Constant1/1 -> Subtract1/1
  angleBtw2DVecs1/1(angle) -> Subtract1/2
  Constant5/1 -> Matrix Multiply2/2

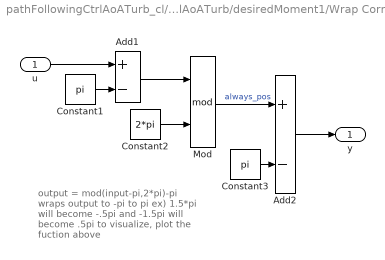
== system pathFollowingCtrlAoATurb_cl/pathFollowingCtrlAoATurb/desiredMoment1/Wrap Correction ==
  note: output = mod(input-pi,2*pi)-pi
      | wraps output to -pi to pi
      |
      | ex) 1.5*pi will become -.5pi
      | 	and -1.5pi will become .5pi
      |
      | to visualize, plot the fuction above
  u : Inport
  Add1 : Sum  Inputs=+-
  Add2 : Sum  Inputs=+-
  Constant1 : Constant  Value=pi
  Constant2 : Constant  Value=2*pi
  Constant3 : Constant  Value=pi
  Mod : Math  Operator=mod  SignedPower=on
  y : Outport  VectorParamsAs1DForOutWhenUnconnected=off
  wires:
  u/1 -> Add1/1
  Constant1/1 -> Add1/2
  Add1/1 -> Mod/1
  Constant2/1 -> Mod/2
  Mod/1 -> Add2/1  "always_pos"
  Constant3/1 -> Add2/2
  Add2/1 -> y/1

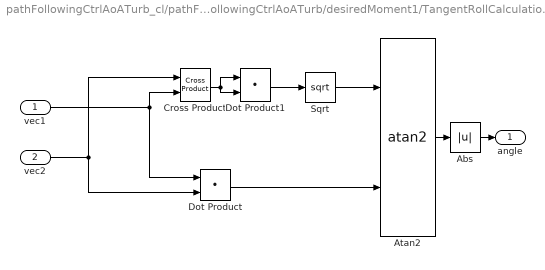
== system pathFollowingCtrlAoATurb_cl/pathFollowingCtrlAoATurb/desiredMoment1/TangentRollCalculation/angleBtw2DVecs1 ==
  vec1 : Inport
  vec2 : Inport  Port=2
  Abs : Abs  SaturateOnIntegerOverflow=off
  Atan2 : Trigonometry  Operator=atan2
  Cross Product : vrlib/Utilities/Cross Product
  Dot Product : DotProduct  OutDataTypeStr=Inherit: Inherit via internal rule
  Dot Product1 : DotProduct  OutDataTypeStr=Inherit: Inherit via internal rule
  Sqrt : Sqrt
  angle : Outport  VectorParamsAs1DForOutWhenUnconnected=off
  wires:
  Atan2/1 -> Abs/1
  vec1/1 -> Dot Product/1, Cross Product/2
  vec2/1 -> Cross Product/1, Dot Product/2
  Cross Product/1 -> Dot Product1/1, Dot Product1/2
  Dot Product/1 -> Atan2/2
  Abs/1 -> angle/1
  Dot Product1/1 -> Sqrt/1
  Sqrt/1 -> Atan2/1
